simulink model "ModulationASK1"  (R2020a)
settings: Solver=ode45  StartTime=0.0  StopTime=750  RelTol=1e-3
libraries: commrandsrc2 x1, dspsrcs4 x1
settings Model: Creator=Administrateur  LastModifiedBy=J-MENTION
settings DataIOCC: LimitDataPoints=on  SaveFormat=Array  SignalLoggingSaveFormat=ModelDataLogs  ReturnWorkspaceOutputs=off
settings OptimizationCC: ExpressionDepthLimit=2147483647  InitFltsAndDblsToZero=on  LifeSpan=inf
settings DebuggingCC: UnderspecifiedInitializationDetection=Classic  MergeDetectMultiDrivingBlocksExec=none  SolverPrmCheckMsg=warning  FcnCallInpInsideContextMsg=warning  StateNameClashWarn=warning  SFUnexpectedBacktrackingDiag=warning  SFNoUnconditionalDefaultTransitionDiag=warning  SFExecutionAtInitializationDiag=none  ArithmeticOperatorsInVariantConditions=warning
settings HardwareCC: ProdBitPerPointer=32  ProdBitPerSizeT=32  ProdBitPerPtrDiffT=32  ProdLargestAtomicFloat=None  ProdIntDivRoundTo=Undefined  ProdEndianess=Unspecified  ProdWordSize=32  ProdHWDeviceType=32-bit Generic
settings ModelReferenceCC: PropagateSignalLabelsOutOfModel=off
settings SFSimCC: SimUseLocalCustomCode=off  CustomCodeUndefinedFunction=UseInterfaceOnly
settings RTWCC: RTWUseLocalCustomCode=off
settings CodeAppCC: StateflowObjectComments=on
settings GRTTargetCC: TargetLangStandard=C89/C90 (ANSI)  CombineOutputUpdateFcns=off  GRTInterface=on
settings ConfigComp: CovMetricSettings=dw  CovHtmlReporting=on  CovSaveCumulativeToWorkspaceVar=on  CovSaveSingleToWorkspaceVar=on  CovExternalEMLEnable=off

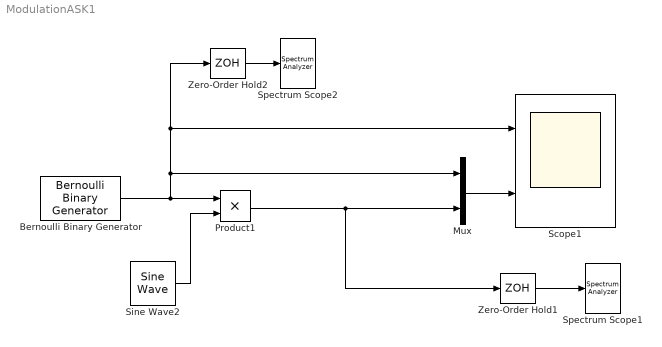
== system ModulationASK1 ==
  Bernoulli Binary Generator : commrandsrc2/Bernoulli Binary Generator  P=0.5  seed=61  Ts=1  frameBased=off  sampPerFrame=1  orient=off  outDataType=double
      settings: SourceProductBaseCode=CM
  Mux : Mux  Inputs=2
  Product1 : Product  RndMeth=Zero
  Scope1 : Scope  NumInputPorts=2
  Sine Wave2 : dspsrcs4/Sine Wave  Amplitude=1  Frequency=5  Phase=0  SampleMode=Discrete  OutComplex=Real  CompMethod=Trigonometric fcn  TableSize=Speed  SampleTime=1/100  SamplesPerFrame=1  ResetState=Restart at time zero  OutputFrames=on  dataType=double  wordLen=16  udDataType=sfix(16)  fracBitsMode=Best precision  numFracBits=15  OutDataTypeStr=double  LastOutDataTypeStr=double
  Spectrum Scope1 : SpectrumAnalyzer
  Spectrum Scope2 : SpectrumAnalyzer
  Zero-Order Hold1 : ZeroOrderHold  SampleTime=1/50
  Zero-Order Hold2 : ZeroOrderHold  SampleTime=1/50
  wires:
  Bernoulli Binary Generator/1 -> Product1/1, Mux/1, Zero-Order Hold2/1, Scope1/1
  Sine Wave2/1 -> Product1/2
  Product1/1 -> Mux/2, Zero-Order Hold1/1
  Zero-Order Hold1/1 -> Spectrum Scope1/1
  Zero-Order Hold2/1 -> Spectrum Scope2/1
  Mux/1 -> Scope1/2
